simulink model "heli_simulator_day3"  (R2025a)
settings: Solver=ode23s  StartTime=0.0  StopTime=60  FixedStep=0.002  MaxStep=0.002  RelTol=1e-3
values from neighbouring files (symbols this model uses):
  K = dlqr(A,B,Q,R)    [init_simulator_day3.m]
  K_ed = 2*d_e*sqrt(K_ep/K_3)    [init_simulator_day3.m]
  K_ei = K_ep*0.1    (= 0.303465851172)    [init_simulator_day3.m]
  K_ep = w_e^2/K_3    (= 3.03465851172)    [init_simulator_day3.m]
  K_pd = 2*d_p*sqrt(K_pp/K_1)    [init_simulator_day3.m]
  K_pp = w_p^2/K_1    (= 5.14304587156)    [init_simulator_day3.m]
  Vd_ff = V_d_eq    (= 0)    [init_simulator_day3.m]
  Vs_ff = V_s_eq    (= 6.87)    [init_simulator_day3.m]
  x0_sim = [pi, -deg2rad(30),0,0,0,0]'    [init_simulator_day3.m]
libraries: simulink_extras x4
settings Model: Creator=joakira  LastModifiedBy=mathi
settings SolverCC: AlgebraicLoopSolver=TrustRegion
settings DebuggingCC: UnconnectedInputMsg=warning  UnconnectedOutputMsg=warning  UnconnectedLineMsg=warning
settings ModelReferenceCC: EnableRefExpFcnMdlSchedulingChecks=on
settings RTWCC: GPUComputeCapability=3.5  DLArmComputeVersion=19.05

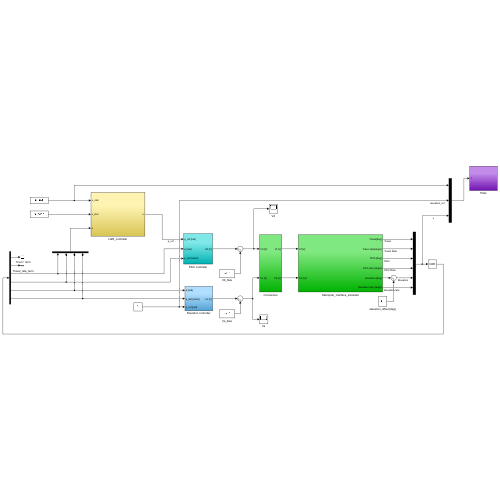
[thumbnail: Simulink's stored preview of the top-level diagram]
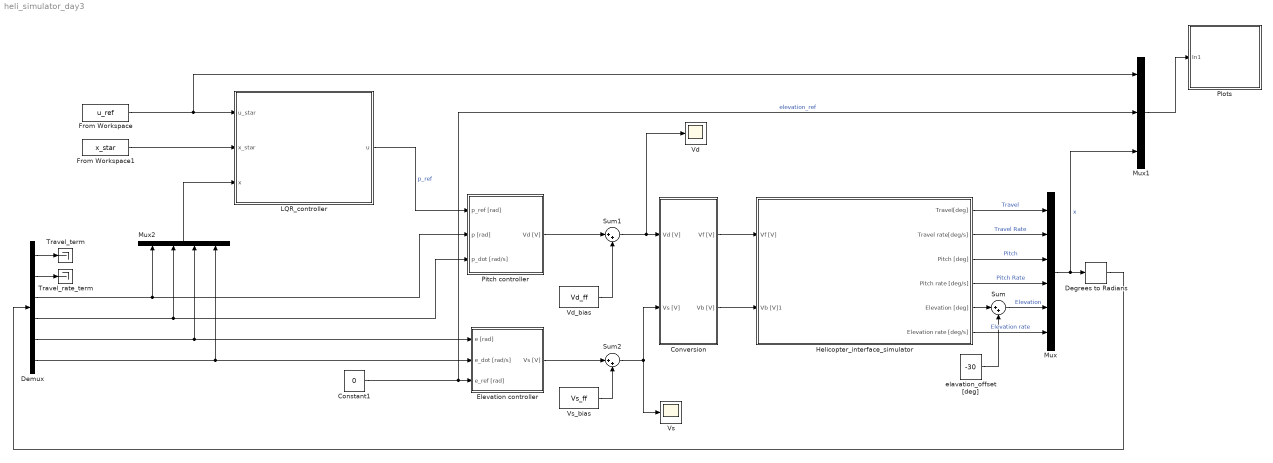
== system heli_simulator_day3 ==
  Constant1 : Constant  Value=0
  Conversion : Subsystem
  Degrees to Radians : simulink_extras/Transformations/Degrees to Radians
  Demux : Demux  Outputs=6
  Elevation controller : Subsystem
  From Workspace : FromWorkspace  VariableName=u_ref
  From Workspace1 : FromWorkspace  VariableName=x_star
  Helicopter_interface_simulator : Subsystem
  LQR_controller : Subsystem
  Mux : Mux  Inputs=6
  Mux1 : Mux  Inputs=3
  Mux2 : Mux
  Pitch controller : Subsystem
  Plots : Subsystem
  Sum : Sum  Inputs=|++
  Sum1 : Sum  Inputs=|++
  Sum2 : Sum  Inputs=|++
  Travel_rate_term : Terminator
  Travel_term : Terminator
  Vd : Scope
      settings: ActiveDisplayYMinimum=-6E-16  ActiveDisplayYMaximum=6E-16
  Vd_bias : Constant  Value=Vd_ff
  Vs : Scope
      settings: ActiveDisplayYMinimum=5.91361  ActiveDisplayYMaximum=8.74176  DataLoggingVariableName=ScopeData3
  Vs_bias : Constant  Value=Vs_ff
  elavation_offset [deg] : Constant  Value=-30
  wires:
  Helicopter_interface_simulator/1(Travel[deg]) -> Mux/1  "Travel"
  Vd_bias/1 -> Sum1/2
  Helicopter_interface_simulator/6(Elevation rate [deg/s]) -> Mux/6  "Elevation rate"
  Sum2/1 -> Conversion/2(Vs [V]), Vs/1
  Helicopter_interface_simulator/5(Elevation [deg]) -> Sum/1
  Demux/4 -> Pitch controller/3(p_dot [rad/s]), Mux2/2
  Elevation controller/1(Vs [V]) -> Sum2/1
  Sum1/1 -> Vd/1, Conversion/1(Vd [V])
  Constant1/1 -> Elevation controller/3(e_ref [rad]), Mux1/2  "elevation_ref"
  Vs_bias/1 -> Sum2/2
  Mux/1 -> Mux1/3, Degrees to Radians/1  "x"
  Degrees to Radians/1 -> Demux/1
  Demux/6 -> Elevation controller/2(e_dot [rad/s]), Mux2/4
  Demux/5 -> Elevation controller/1(e [rad]), Mux2/3
  Helicopter_interface_simulator/4(Pitch rate [deg/s]) -> Mux/4  "Pitch Rate"
  Helicopter_interface_simulator/2(Travel rate[deg/s]) -> Mux/2  "Travel Rate"
  Helicopter_interface_simulator/3(Pitch [deg]) -> Mux/3  "Pitch"
  Demux/2 -> Travel_rate_term/1
  Demux/1 -> Travel_term/1
  Sum/1 -> Mux/5  "Elevation"
  elavation_offset [deg]/1 -> Sum/2
  Demux/3 -> Mux2/1, Pitch controller/2(p [rad])
  Pitch controller/1(Vd [V]) -> Sum1/1
  Conversion/1(Vf [V]) -> Helicopter_interface_simulator/1(Vf [V])
  Conversion/2(Vb [V]) -> Helicopter_interface_simulator/2(Vb [V]1)
  Mux1/1 -> Plots/1(In1)
  From Workspace/1 -> Mux1/1, LQR_controller/1(u_star)
  From Workspace1/1 -> LQR_controller/2(x_star)
  LQR_controller/1(u) -> Pitch controller/1(p_ref [rad])  "p_ref"
  Mux2/1 -> LQR_controller/3(x)

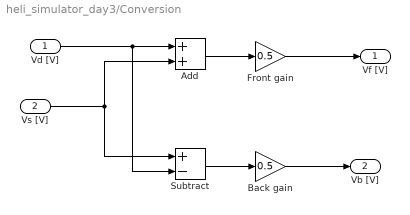
== system heli_simulator_day3/Conversion ==
  Vd [V] : Inport
  Vs [V] : Inport  Port=2
  Add : Sum
  Back gain : Gain  Gain=0.5
  Front gain : Gain  Gain=0.5
  Subtract : Sum  Inputs=+-
  Vf [V] : Outport
  Vb [V] : Outport  Port=2
  wires:
  Vd [V]/1 -> Subtract/2, Add/1
  Vs [V]/1 -> Subtract/1, Add/2
  Subtract/1 -> Back gain/1
  Back gain/1 -> Vb [V]/1
  Add/1 -> Front gain/1
  Front gain/1 -> Vf [V]/1

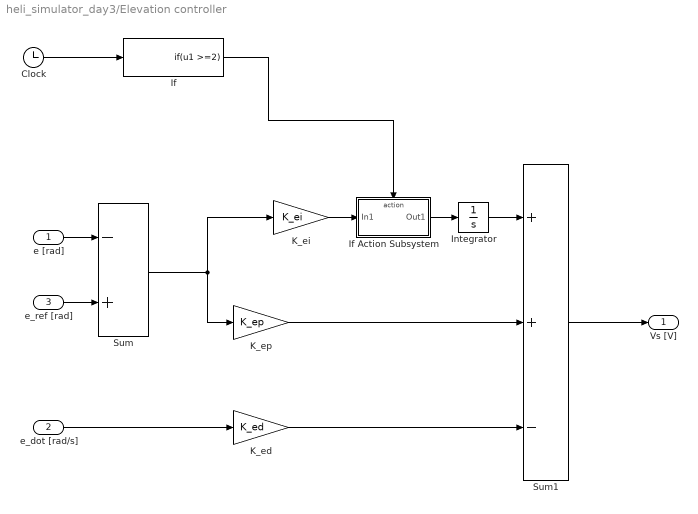
== system heli_simulator_day3/Elevation controller ==
  e [rad] : Inport
  e_dot [rad/s] : Inport  Port=2
  e_ref [rad] : Inport  Port=3
  Clock : Clock
  If : If  IfExpression=u1 >=2  ShowElse=off
  If Action Subsystem : Subsystem  TreatAsAtomicUnit=on
  Integrator : Integrator  LimitOutput=on
  K_ed : Gain  Gain=K_ed  SaturateOnIntegerOverflow=on  OutDataTypeStr=Inherit: Same as input  ParamDataTypeStr=Inherit: Same as input
  K_ei : Gain  Gain=K_ei  SaturateOnIntegerOverflow=on  OutDataTypeStr=Inherit: Same as input  ParamDataTypeStr=Inherit: Same as input
  K_ep : Gain  Gain=K_ep  SaturateOnIntegerOverflow=on  OutDataTypeStr=Inherit: Same as input  ParamDataTypeStr=Inherit: Same as input
  Sum : Sum  Inputs=-+  InputSameDT=on  SaturateOnIntegerOverflow=on  OutDataTypeStr=Inherit: Same as first input
  Sum1 : Sum  Inputs=++-  InputSameDT=on  SaturateOnIntegerOverflow=on  OutDataTypeStr=Inherit: Same as first input
  Vs [V] : Outport  InitialOutput=0
  wires:
  Integrator/1 -> Sum1/1
  e_ref [rad]/1 -> Sum/2
  If/1 -> If Action Subsystem/Action
  Clock/1 -> If/1
  K_ei/1 -> If Action Subsystem/1(In1)
  e_dot [rad/s]/1 -> K_ed/1
  If Action Subsystem/1(Out1) -> Integrator/1
  K_ed/1 -> Sum1/3
  Sum1/1 -> Vs [V]/1
  e [rad]/1 -> Sum/1
  K_ep/1 -> Sum1/2
  Sum/1 -> K_ep/1, K_ei/1

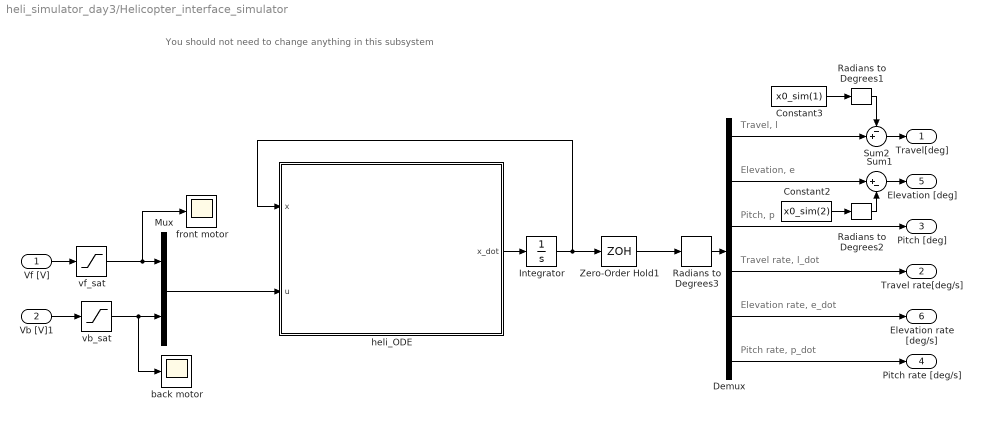
== system heli_simulator_day3/Helicopter_interface_simulator ==
  note: You should not need to change anything in this subsystem
  note: Pitch, p
  note: Elevation rate, e_dot
  note: Travel, l
  note: Elevation, e
  note: Travel rate, l_dot
  note: Pitch rate, p_dot
  Vf [V] : Inport
  Vb [V]1 : Inport  Port=2
  Constant2 : Constant  Value=x0_sim(2)
  Constant3 : Constant  Value=x0_sim(1)
  Demux : Demux  Outputs=6
  Integrator : Integrator  InitialCondition=x0_sim
  Mux : Mux  Inputs=2
  Radians to Degrees1 : simulink_extras/Transformations/Radians to Degrees
  Radians to Degrees2 : simulink_extras/Transformations/Radians to Degrees
  Radians to Degrees3 : simulink_extras/Transformations/Radians to Degrees
  Sum1 : Sum  Inputs=|+-
  Sum2 : Sum  Inputs=-+|
  Zero-Order Hold1 : ZeroOrderHold  SampleTime=0.058
  back motor : Scope
      settings: ActiveDisplayYMinimum=0.78479  ActiveDisplayYMaximum=0.784803  DataLoggingVariableName=ScopeData4
  front motor : Scope
      settings: ActiveDisplayYMinimum=3.08761  ActiveDisplayYMaximum=5.49145  DataLoggingVariableName=ScopeData3
  heli_ODE : MATLAB Function  TreatAsAtomicUnit=on
  vb_sat : Saturate  UpperLimit=5  LowerLimit=-5
  vf_sat : Saturate  UpperLimit=5  LowerLimit=-5
  Travel[deg] : Outport
  Travel rate[deg/s] : Outport  Port=2
  Pitch [deg] : Outport  Port=3
  Pitch rate [deg/s] : Outport  Port=4
  Elevation [deg] : Outport  Port=5
  Elevation rate [deg/s] : Outport  Port=6
  wires:
  Sum1/1 -> Elevation [deg]/1
  Demux/2 -> Sum1/1
  Mux/1 -> heli_ODE/2(u)
  Radians to Degrees3/1 -> Demux/1
  Demux/6 -> Pitch rate [deg/s]/1
  Demux/5 -> Elevation rate [deg/s]/1
  Demux/4 -> Travel rate[deg/s]/1
  Demux/3 -> Pitch [deg]/1
  heli_ODE/1(x_dot) -> Integrator/1
  Vf [V]/1 -> vf_sat/1
  Demux/1 -> Sum2/2
  Sum2/1 -> Travel[deg]/1
  Vb [V]1/1 -> vb_sat/1
  Zero-Order Hold1/1 -> Radians to Degrees3/1
  Integrator/1 -> Zero-Order Hold1/1, heli_ODE/1(x)
  vf_sat/1 -> front motor/1, Mux/1
  vb_sat/1 -> back motor/1, Mux/2
  Constant3/1 -> Radians to Degrees1/1
  Radians to Degrees1/1 -> Sum2/1
  Constant2/1 -> Radians to Degrees2/1
  Radians to Degrees2/1 -> Sum1/2

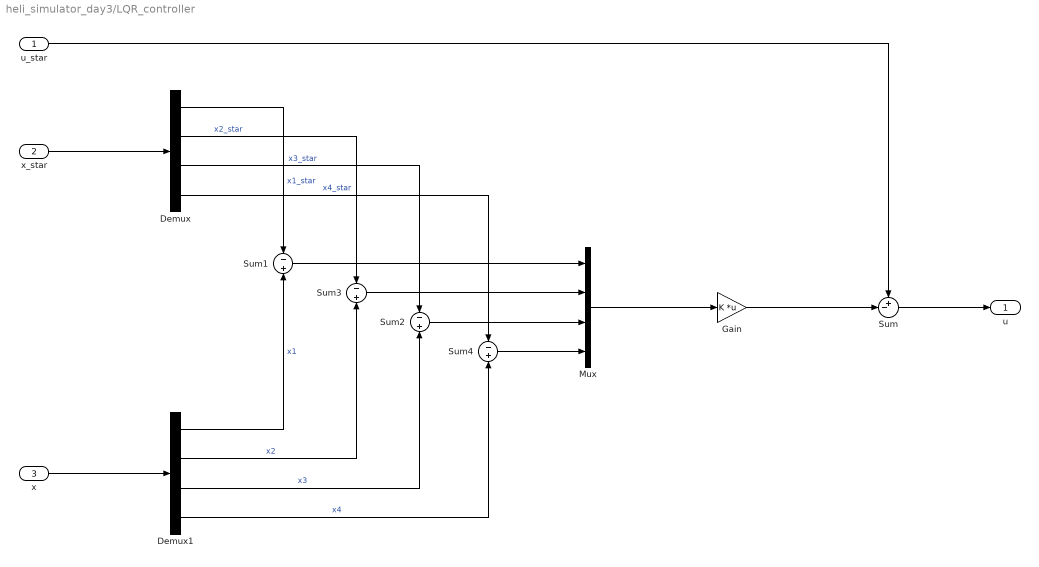
== system heli_simulator_day3/LQR_controller ==
  u_star : Inport
  x_star : Inport  Port=2
  x : Inport  Port=3
  Demux : Demux
  Demux1 : Demux
  Gain : Gain  Gain=K  Multiplication=Matrix(K*u) (u vector)
  Mux : Mux
  Sum : Sum  Inputs=+-|
  Sum{1..4} (4 alike) : Sum  Inputs=-+
  u : Outport
  wires:
  x_star/1 -> Demux/1
  x/1 -> Demux1/1
  Mux/1 -> Gain/1
  Gain/1 -> Sum/2
  Sum/1 -> u/1
  u_star/1 -> Sum/1
  Sum1/1 -> Mux/1
  Sum3/1 -> Mux/2
  Sum2/1 -> Mux/3
  Sum4/1 -> Mux/4
  Demux/1 -> Sum1/1  "x1_star"
  Demux1/1 -> Sum1/2  "x1"
  Demux/2 -> Sum3/1  "x2_star"
  Demux1/2 -> Sum3/2  "x2"
  Demux/3 -> Sum2/1  "x3_star"
  Demux1/3 -> Sum2/2  "x3"
  Demux/4 -> Sum4/1  "x4_star"
  Demux1/4 -> Sum4/2  "x4"

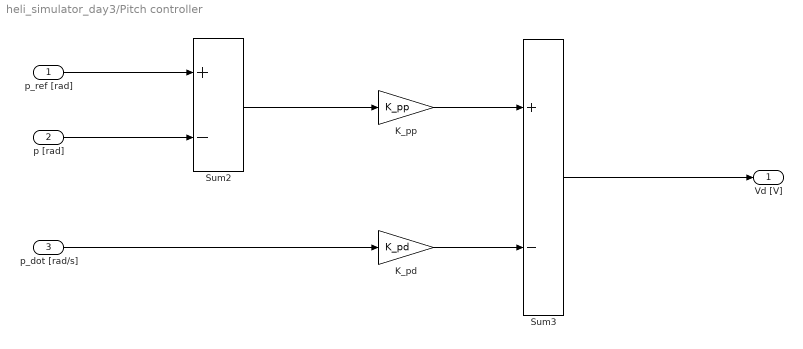
== system heli_simulator_day3/Pitch controller ==
  p_ref [rad] : Inport
  p [rad] : Inport  Port=2
  p_dot [rad/s] : Inport  Port=3
  K_pd : Gain  Gain=K_pd  SaturateOnIntegerOverflow=on  OutDataTypeStr=Inherit: Same as input  ParamDataTypeStr=Inherit: Same as input
  K_pp : Gain  Gain=K_pp  SaturateOnIntegerOverflow=on  OutDataTypeStr=Inherit: Same as input  ParamDataTypeStr=Inherit: Same as input
  Sum2 : Sum  Inputs=+-  InputSameDT=on  SaturateOnIntegerOverflow=on  OutDataTypeStr=Inherit: Same as first input
  Sum3 : Sum  Inputs=+-  InputSameDT=on  SaturateOnIntegerOverflow=on  OutDataTypeStr=Inherit: Same as first input
  Vd [V] : Outport  InitialOutput=0
  wires:
  p_ref [rad]/1 -> Sum2/1
  p [rad]/1 -> Sum2/2
  p_dot [rad/s]/1 -> K_pd/1
  K_pp/1 -> Sum3/1
  Sum2/1 -> K_pp/1
  K_pd/1 -> Sum3/2
  Sum3/1 -> Vd [V]/1

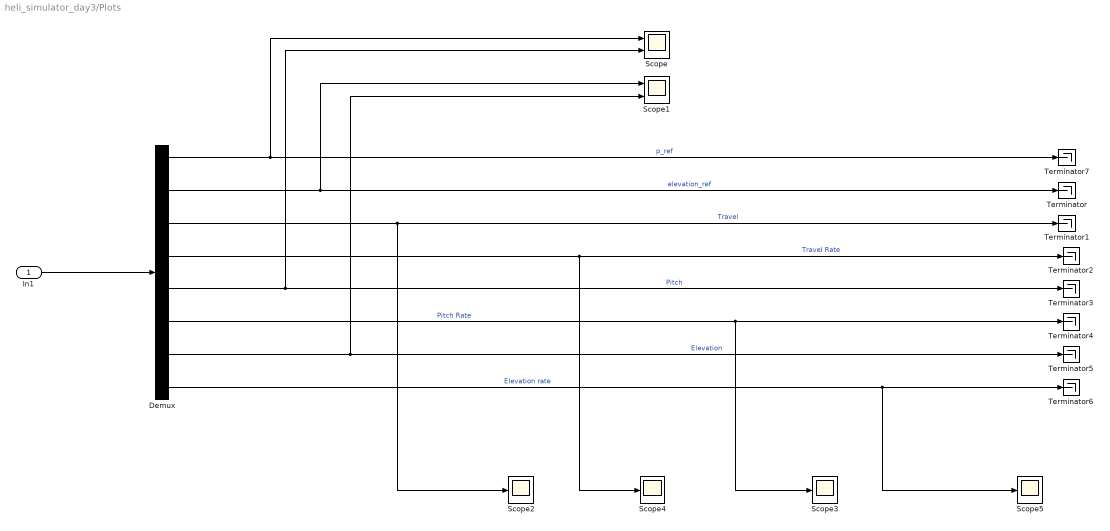
== system heli_simulator_day3/Plots ==
  In1 : Inport
  Demux : Demux  Outputs=8
  Scope : Scope  NumInputPorts=2
      settings: ActiveDisplayYMinimum=-31.449753607517479  ActiveDisplayYMaximum=30.476083828658773
  Scope1 : Scope  NumInputPorts=2
      settings: ActiveDisplayYMinimum=-33.914524543341564  ActiveDisplayYMaximum=5.2307208900740942  DataLoggingVariableName=ScopeData2
  Scope{2..5} (4 alike) : Scope
      Scope2 settings: ActiveDisplayYMinimum=-139.83052592503407  ActiveDisplayYMaximum=1258.4747333253069  DataLoggingVariableName=ScopeData5
      Scope3 settings: ActiveDisplayYMinimum=-23.327670549507012  ActiveDisplayYMaximum=24.152573157545977  DataLoggingVariableName=ScopeData6
      Scope4 settings: ActiveDisplayYMinimum=-4.8499436525394932  ActiveDisplayYMaximum=43.649492872855447  DataLoggingVariableName=ScopeData7
      Scope5 settings: ActiveDisplayYMinimum=-1.1330592728772084  ActiveDisplayYMaximum=9.6374966506825555  DataLoggingVariableName=ScopeData8
  Terminator{,1..7} (8 alike) : Terminator
  wires:
  In1/1 -> Demux/1
  Demux/2 -> Terminator/1, Scope1/1  "elevation_ref"
  Demux/8 -> Scope5/1, Terminator6/1  "Elevation rate"
  Demux/4 -> Terminator2/1, Scope4/1  "Travel Rate"
  Demux/3 -> Scope2/1, Terminator1/1  "Travel"
  Demux/6 -> Terminator4/1, Scope3/1  "Pitch Rate"
  Demux/7 -> Terminator5/1, Scope1/2  "Elevation"
  Demux/5 -> Terminator3/1, Scope/2  "Pitch"
  Demux/1 -> Terminator7/1, Scope/1  "p_ref"

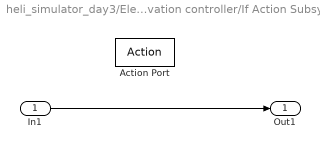
== system heli_simulator_day3/Elevation controller/If Action Subsystem ==
  In1 : Inport
  Action Port : ActionPort  ActionPortLabel=if(u1 >=2)
  Out1 : Outport
  wires:
  In1/1 -> Out1/1

== matlab function heli_simulator_day3/Helicopter_interface_simulator/heli_ODE ==
  data: x input; u input; x_dot output
function x_dot = helicopter_ODE(x, u)
% x = [l, e, p, l_dot, e_dot, p_dot]
% u = [V_f, V_b]
coder.extrinsic('xdot_c'); 
x_dot = zeros(6,1);
x_dot = xdot_c('xdot_fun', x, u);
